simulink model "Q4"  (R2021b)
settings: Solver=ode45  StartTime=0.0  StopTime=5  RelTol=1e-3  EnableMultiTasking=on
values from neighbouring files (symbols this model uses):
  a = 10    [Q4.m]
  b = 11    [Q4.m]
  J = 1.92e-3    (= 0.00192)    [Q4.m]
  L_A = 6.82e-3    (= 0.00682)    [Q4.m]
  M_F = 0.36e-3    (= 0.00036)    [Q4.m]
  R_A = 1.52    [Q4.m]
  sai = 0.33    [Q4.m]
settings Model: Creator=Admin  LastModifiedBy=user
settings SolverCC: AlgebraicLoopSolver=TrustRegion
settings DataIOCC: LimitDataPoints=on  SaveFormat=Array  ReturnWorkspaceOutputs=off
settings OptimizationCC: ExpressionDepthLimit=2147483647  LifeSpan=inf
settings DebuggingCC: UnderspecifiedInitializationDetection=Classic  MergeDetectMultiDrivingBlocksExec=none  SolverPrmCheckMsg=warning  StateNameClashWarn=warning  SFUnexpectedBacktrackingDiag=warning  SFNoUnconditionalDefaultTransitionDiag=warning  SFExecutionAtInitializationDiag=none  SFMachineParentedDataDiag=warning  ArithmeticOperatorsInVariantConditions=warning
settings HardwareCC: ProdBitPerPointer=32  ProdBitPerSizeT=32  ProdBitPerPtrDiffT=32  ProdLargestAtomicFloat=None  ProdIntDivRoundTo=Undefined  ProdEndianess=Unspecified  ProdWordSize=32  ProdHWDeviceType=32-bit Generic
settings ModelReferenceCC: PropagateSignalLabelsOutOfModel=off
settings SFSimCC: SimUseLocalCustomCode=off  CustomCodeUndefinedFunction=UseInterfaceOnly
settings RTWCC: RTWUseLocalCustomCode=off
settings CodeAppCC: StateflowObjectComments=on
settings GRTTargetCC: TargetLangStandard=C89/C90 (ANSI)
settings ConfigComp: CovMetricSettings=dw  CovSaveCumulativeToWorkspaceVar=on  CovSaveSingleToWorkspaceVar=on  CovExternalEMLEnable=off

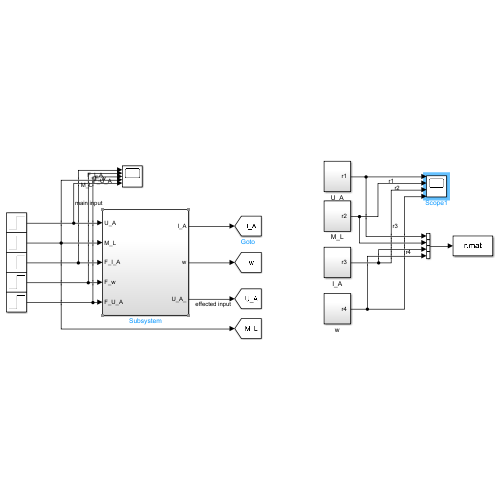
[thumbnail: Simulink's stored preview of the top-level diagram]
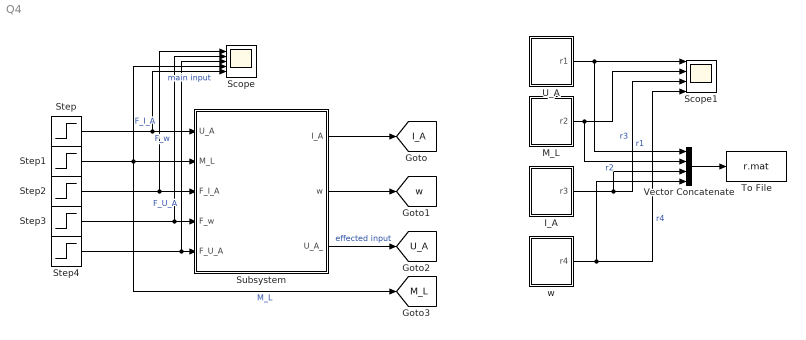
== system Q4 ==
  I_A : Subsystem
  M_L : Subsystem
  Scope : Scope  NumInputPorts=5
  Scope1 : Scope  NumInputPorts=4
  Step{,1..3} (4 alike) : Step  Time=0  After=0  SampleTime=0
  Step4 : Step  Time=2  After=2  SampleTime=0
  Subsystem : Subsystem
  To File : ToFile  Filename=r.mat  SaveFormat=Timeseries
  U_A : Subsystem
  Vector Concatenate : Concatenate  NumInputs=4
  w : Subsystem
  tag scope: I_A=global, M_L=global, U_A=global, w=global
  wires:
  Step/1 -> Scope/5, Subsystem/1(U_A)  "main input"
  Step1/1 -> [M_L], Scope/4, Subsystem/2(M_L)  "M_L"
  Step2/1 -> Scope/1, Subsystem/3(F_I_A)  "F_I_A"
  Step3/1 -> Scope/2, Subsystem/4(F_w)  "F_w"
  Step4/1 -> Scope/3, Subsystem/5(F_U_A)  "F_U_A"
  Subsystem/1(I_A) -> [I_A]
  Subsystem/2(w) -> [w]
  Subsystem/3(U_A_) -> [U_A]  "effected input"
  U_A/1("r1 ") -> Vector Concatenate/1, Scope1/1  "r1"
  I_A/1("r3 ") -> Vector Concatenate/3, Scope1/3  "r3"
  w/1("r4 ") -> Vector Concatenate/4, Scope1/4  "r4"
  M_L/1("r2 ") -> Vector Concatenate/2, Scope1/2  "r2"
  Vector Concatenate/1 -> To File/1

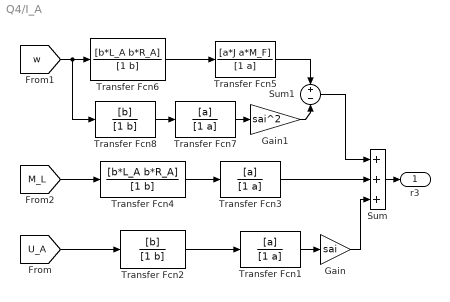
== system Q4/I_A ==
  Gain : Gain  Gain=sai
  Gain1 : Gain  Gain=sai^2
  Sum : Sum  Inputs=+++
  Sum1 : Sum  Inputs=+-
  Transfer Fcn1 : TransferFcn  Numerator=[a]  Denominator=[1 a]
  Transfer Fcn2 : TransferFcn  Numerator=[b]  Denominator=[1 b]
  Transfer Fcn3 : TransferFcn  Numerator=[a]  Denominator=[1 a]
  Transfer Fcn4 : TransferFcn  Numerator=[b*L_A b*R_A]  Denominator=[1 b]
  Transfer Fcn5 : TransferFcn  Numerator=[a*J a*M_F]  Denominator=[1 a]
  Transfer Fcn6 : TransferFcn  Numerator=[b*L_A b*R_A]  Denominator=[1 b]
  Transfer Fcn7 : TransferFcn  Numerator=[a]  Denominator=[1 a]
  Transfer Fcn8 : TransferFcn  Numerator=[b]  Denominator=[1 b]
  "r3 " : Outport
  wires:
  Sum/1 -> "r3 "/1
  Gain/1 -> Sum/3
  Transfer Fcn3/1 -> Sum/2
  [U_A] -> Transfer Fcn2/1
  Transfer Fcn2/1 -> Transfer Fcn1/1
  Transfer Fcn1/1 -> Gain/1
  [M_L] -> Transfer Fcn4/1
  Transfer Fcn4/1 -> Transfer Fcn3/1
  Transfer Fcn6/1 -> Transfer Fcn5/1
  Transfer Fcn5/1 -> Sum1/1
  [w] -> Transfer Fcn8/1, Transfer Fcn6/1
  Transfer Fcn7/1 -> Gain1/1
  Gain1/1 -> Sum1/2
  Transfer Fcn8/1 -> Transfer Fcn7/1
  Sum1/1 -> Sum/1

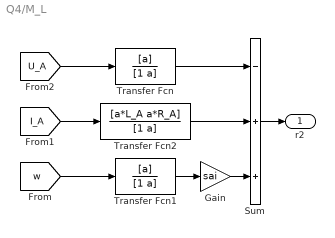
== system Q4/M_L ==
  Gain : Gain  Gain=sai
  Sum : Sum  Inputs=-++
  Transfer Fcn : TransferFcn  Numerator=[a]  Denominator=[1 a]
  Transfer Fcn1 : TransferFcn  Numerator=[a]  Denominator=[1 a]
  Transfer Fcn2 : TransferFcn  Numerator=[a*L_A a*R_A]  Denominator=[1 a]
  "r2 " : Outport
  wires:
  [I_A] -> Transfer Fcn2/1
  Gain/1 -> Sum/3
  Transfer Fcn2/1 -> Sum/2
  Sum/1 -> "r2 "/1
  [U_A] -> Transfer Fcn/1
  Transfer Fcn/1 -> Sum/1
  [w] -> Transfer Fcn1/1
  Transfer Fcn1/1 -> Gain/1

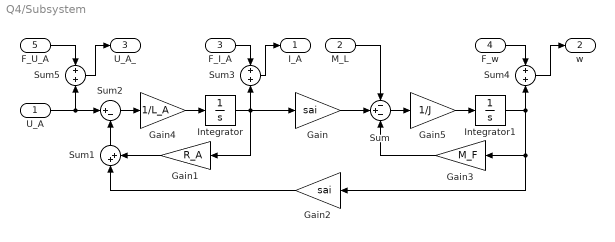
== system Q4/Subsystem ==
  U_A : Inport
  M_L : Inport  Port=2
  F_I_A : Inport  Port=3
  F_w : Inport  Port=4
  F_U_A : Inport  Port=5
  Gain : Gain  Gain=sai
  Gain1 : Gain  Gain=R_A
  Gain2 : Gain  Gain=sai
  Gain3 : Gain  Gain=M_F
  Gain4 : Gain  Gain=1/L_A
  Gain5 : Gain  Gain=1/J
  Integrator : Integrator
  Integrator1 : Integrator
  Sum : Sum  Inputs=-+-
  Sum1 : Sum  Inputs=|++
  Sum2 : Sum  Inputs=|+-
  Sum3 : Sum
  Sum4 : Sum
  Sum5 : Sum
  I_A : Outport
  w : Outport  Port=2
  U_A_ : Outport  Port=3
  wires:
  Gain1/1 -> Sum1/2
  M_L/1 -> Sum/1
  F_I_A/1 -> Sum3/1
  F_w/1 -> Sum4/1
  Integrator1/1 -> Sum4/2, Gain2/1, Gain3/1
  Sum3/1 -> I_A/1
  Sum2/1 -> Gain4/1
  Gain2/1 -> Sum1/1
  Sum/1 -> Gain5/1
  Gain5/1 -> Integrator1/1
  Sum1/1 -> Sum2/2
  Gain4/1 -> Integrator/1
  U_A/1 -> Sum2/1, Sum5/2
  Sum4/1 -> w/1
  Integrator/1 -> Gain/1, Gain1/1, Sum3/2
  Gain/1 -> Sum/2
  Gain3/1 -> Sum/3
  F_U_A/1 -> Sum5/1
  Sum5/1 -> U_A_/1

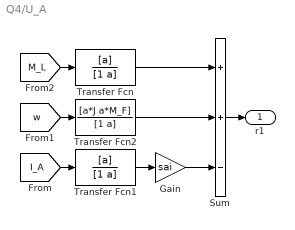
== system Q4/U_A ==
  Gain : Gain  Gain=sai
  Sum : Sum  Inputs=++-
  Transfer Fcn : TransferFcn  Numerator=[a]  Denominator=[1 a]
  Transfer Fcn1 : TransferFcn  Numerator=[a]  Denominator=[1 a]
  Transfer Fcn2 : TransferFcn  Numerator=[a*J a*M_F]  Denominator=[1 a]
  "r1 " : Outport
  wires:
  Sum/1 -> "r1 "/1
  Gain/1 -> Sum/3
  [w] -> Transfer Fcn2/1
  [M_L] -> Transfer Fcn/1
  Transfer Fcn/1 -> Sum/1
  [I_A] -> Transfer Fcn1/1
  Transfer Fcn1/1 -> Gain/1
  Transfer Fcn2/1 -> Sum/2

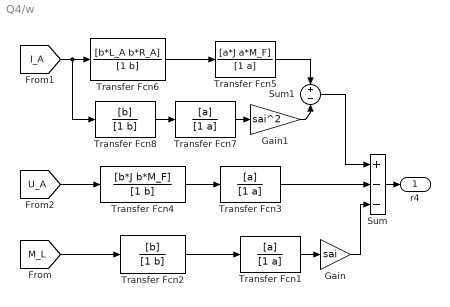
== system Q4/w ==
  Gain : Gain  Gain=sai
  Gain1 : Gain  Gain=sai^2
  Sum : Sum  Inputs=+--
  Sum1 : Sum  Inputs=+-
  Transfer Fcn1 : TransferFcn  Numerator=[a]  Denominator=[1 a]
  Transfer Fcn2 : TransferFcn  Numerator=[b]  Denominator=[1 b]
  Transfer Fcn3 : TransferFcn  Numerator=[a]  Denominator=[1 a]
  Transfer Fcn4 : TransferFcn  Numerator=[b*J b*M_F]  Denominator=[1 b]
  Transfer Fcn5 : TransferFcn  Numerator=[a*J a*M_F]  Denominator=[1 a]
  Transfer Fcn6 : TransferFcn  Numerator=[b*L_A b*R_A]  Denominator=[1 b]
  Transfer Fcn7 : TransferFcn  Numerator=[a]  Denominator=[1 a]
  Transfer Fcn8 : TransferFcn  Numerator=[b]  Denominator=[1 b]
  "r4 " : Outport
  wires:
  Sum/1 -> "r4 "/1
  Gain/1 -> Sum/3
  Transfer Fcn3/1 -> Sum/2
  [M_L] -> Transfer Fcn2/1
  Transfer Fcn2/1 -> Transfer Fcn1/1
  Transfer Fcn1/1 -> Gain/1
  [U_A] -> Transfer Fcn4/1
  Transfer Fcn4/1 -> Transfer Fcn3/1
  Transfer Fcn6/1 -> Transfer Fcn5/1
  Transfer Fcn5/1 -> Sum1/1
  [I_A] -> Transfer Fcn8/1, Transfer Fcn6/1
  Transfer Fcn7/1 -> Gain1/1
  Gain1/1 -> Sum1/2
  Transfer Fcn8/1 -> Transfer Fcn7/1
  Sum1/1 -> Sum/1
